simulink model "DroneOptimalPlanning"  (R2020b)
settings: Solver=FixedStepAuto  StartTime=0.0  StopTime=Ttot  RelTol=1e-3
values from neighbouring files (symbols this model uses):
  A = eval(A)    [Pianificazione1.m]
  A_d_fe = Ts*A + eye(size(A,1))    [Pianificazione1.m]
  A_d_zoh = sys_d_zoh.a    [Pianificazione1.m]
  B = eval(B)    [Pianificazione1.m]
  B_d_fe = Ts*B    [Pianificazione1.m]
  B_d_zoh = sys_d_zoh.b    [Pianificazione1.m]
  C = eye(12)    [Pianificazione1.m]
  C_d_fe = C    [Pianificazione1.m]
  C_d_zoh = sys_d_zoh.c    [Pianificazione1.m]
  D = zeros(12,4)    [Pianificazione1.m]
  D_d_fe = D    [Pianificazione1.m]
  D_d_zoh = sys_d_zoh.d    [Pianificazione1.m]
  F_lb = -6/4    (= -1.5)    [Pianificazione1.m]
  F_ub = 2    [Pianificazione1.m]
  Ts = 0.1    [Pianificazione1.m]
  x_0 = [0;0;0;0;0;0;0;0;0;0;0;0]    [Pianificazione1.m]
settings Model: Creator=Tommaso  LastModifiedBy=Tommaso
settings OptimizationCC: DefaultParameterBehavior=Inlined  UseDivisionForNetSlopeComputation=on  GainParamInheritBuiltInType=on  UseFloatMulNetSlope=on  InlineInvariantSignals=on  PassReuseOutputArgsAs=Individual arguments  ZeroExternalMemoryAtStartup=off  ZeroInternalMemoryAtStartup=off  NoFixptDivByZeroProtection=on  EfficientFloat2IntCast=on  LifeSpan=1  OptimizeBlockOrder=speed  DifferentSizesBufferReuse=on  EfficientTunableParamExpr=on
settings DebuggingCC: ParameterTunabilityLossMsg=error
settings HardwareCC: ProdBitPerPointer=32  ProdBitPerSizeT=32  ProdBitPerPtrDiffT=32  ProdLargestAtomicInteger=Long  ProdLargestAtomicFloat=Double  ProdWordSize=32  ProdLongLongMode=on  ProdHWDeviceType=ARM Compatible->ARM Cortex-M
settings SFSimCC: MATLABDynamicMemAlloc=off
settings RTWCC: Description=Embedded Coder  SystemTargetFile=ert.tlc  TemplateMakefile=ert_default_tmf  TargetLang=C++
settings CodeAppCC: ForceParamTrailComments=on  IgnoreCustomStorageClasses=off  OperatorAnnotations=on  SimulinkDataObjDesc=on  SFDataObjDesc=on  CustomSymbolStrGlobalVar=rt$N$M  CustomSymbolStrType=$N$M  CustomSymbolStrFcn=$N$M$F  CustomSymbolStrMacro=$N$M  InsertBlockDesc=on
settings ERTTargetCC: TargetLangStandard=C++03 (ISO)  GenerateSampleERTMain=on  IncludeMdlTerminateFcn=off  CombineSignalStateStructs=on  CodeInterfacePackaging=C++ class  SupportComplex=off  SupportContinuousTime=on  InlinedParameterPlacement=NonHierarchical  RootIOFormat=Structure reference  ERTCustomFileTemplate=example_file_process.tlc  ERTFilePackagingFormat=CompactWithDataFile

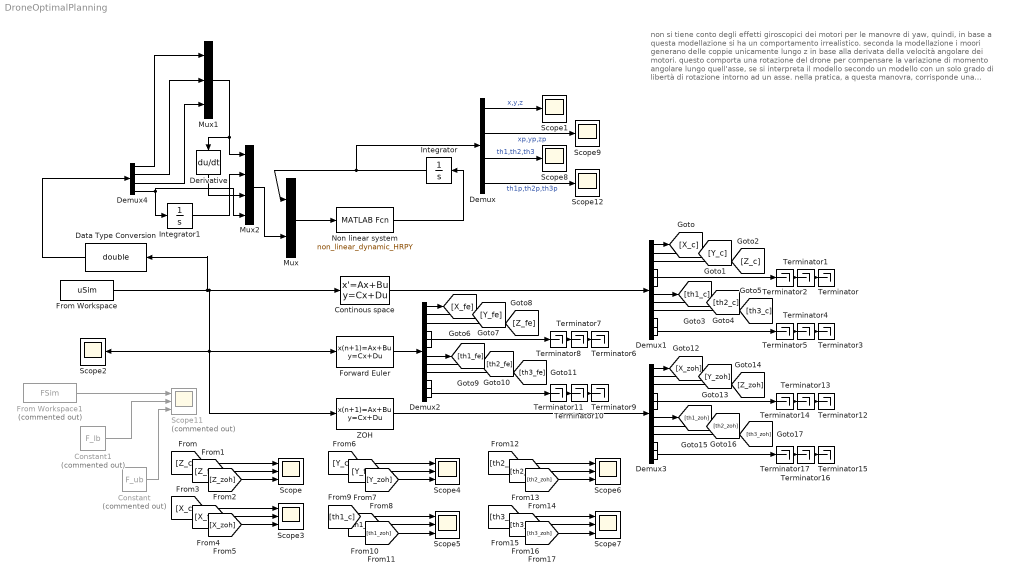
== system DroneOptimalPlanning ==
  note: non si tiene conto degli effetti giroscopici dei motori per le manovre
      | di yaw, quindi, in base a questa modellazione si ha un comportamento irrealistico.
      | seconda la modellazione i moori generano delle coppie unicamente lungo z in base
      | alla derivata della velocità angolare dei motori. questo comporta una rotazione del drone
      | per compensare la variazione di momento angolare lungo quell'asse, se si interpreta il modello secondo un modello con un solo grado di libertà di rotazione intorno ad un asse.
      | nella pratica, a questa manovra, corrisponde una variazione del momento angolare dei motori a cui si accompagna un effetto giroscopico. questi aspetti non sono stati
      | approfonditi. Per incldere quesi aspetti nella modellazione sarebbe necessario modellare
      | la dinamica dei motori e considerare che questi siano montati sul riferimento body
      | a quel punto subentrebbero nelle equazioni degli accoppiamenti tra omegab_x
      | e omegam_z
      | Ho modellato solo l'effetto giroscopico del drone come oggetto nello spazio
      | ho trascurato l'effetto giroscopico dei motori, che è nullo per tutte le manovre
      | ma non per l'imbardata
  Constant : Constant  Commented=on  Value=F_ub
  Constant1 : Constant  Commented=on  Value=F_lb
  Continous space : StateSpace  A=A  B=B  C=C  D=D  InitialCondition=x_0
  Data Type Conversion : DataTypeConversion  OutDataTypeStr=double
  Demux : Demux
  Demux1 : Demux  Outputs=12
  Demux2 : Demux  Outputs=12
  Demux3 : Demux  Outputs=12
  Demux4 : Demux
  Derivative : Derivative
  Forward Euler : DiscreteStateSpace  A=A_d_fe  B=B_d_fe  C=C_d_fe  D=D_d_fe  InitialCondition=x_0  SampleTime=Ts
  From Workspace : FromWorkspace  VariableName=uSim  SampleTime=Ts  OutputAfterFinalValue=Holding final value
  From Workspace1 : FromWorkspace  Commented=on  VariableName=FSim  SampleTime=Ts  OutputAfterFinalValue=Holding final value
  Integrator : Integrator  InitialCondition=x_0  LimitOutput=on  UpperSaturationLimit=10^6  LowerSaturationLimit=-10^6
  Integrator1 : Integrator
  Mux : Mux  Inputs=2
  Mux1 : Mux  Inputs=3
  Mux2 : Mux
  Non linear system : MATLABFcn  MATLABFcn=non_linear_dynamic_HRPY
  Scope{,3..7} (6 alike) : Scope  NumInputPorts=3
  Scope{1..2,8..9,12} (5 alike) : Scope
  Scope11 : Scope  Commented=on  NumInputPorts=3
  Terminator{,1..17} (18 alike) : Terminator
  ZOH : DiscreteStateSpace  A=A_d_zoh  B=B_d_zoh  C=C_d_zoh  D=D_d_zoh  InitialCondition=x_0  SampleTime=Ts
  wires:
  From Workspace/1 -> Data Type Conversion/1, Continous space/1, Scope2/1, ZOH/1, Forward Euler/1
  Mux/1 -> Non linear system/1
  Integrator/1 -> Demux/1, Mux/1
  Non linear system/1 -> Integrator/1
  Continous space/1 -> Demux1/1
  Forward Euler/1 -> Demux2/1
  Demux/1 -> Scope1/1  "x,y,z"
  Demux/3 -> Scope8/1  "th1,th2,th3"
  Demux4/1 -> Mux1/1
  Demux4/2 -> Mux1/2
  Demux4/3 -> Mux1/3
  Demux4/4 -> Mux2/4, Integrator1/1
  Integrator1/1 -> Mux2/2
  Mux1/1 -> Derivative/1, Mux2/1
  Derivative/1 -> Mux2/3
  Mux2/1 -> Mux/2
  Demux/2 -> Scope9/1  "xp,yp,zp"
  From Workspace1/1 -> Scope11/1
  Constant1/1 -> Scope11/2
  Constant/1 -> Scope11/3
  Data Type Conversion/1 -> Demux4/1
  Demux/4 -> Scope12/1  "th1p,th2p,th3p"
  Demux1/1 -> [X_c]
  Demux1/2 -> [Y_c]
  Demux1/3 -> [Z_c]
  Demux1/7 -> [th1_c]
  Demux1/8 -> [th2_c]
  Demux1/9 -> [th3_c]
  Demux1/5 -> Terminator1/1
  Demux1/6 -> Terminator/1
  Demux1/4 -> Terminator2/1
  [Z_c] -> Scope/1
  [Z_fe] -> Scope/2
  [Z_zoh] -> Scope/3
  [X_c] -> Scope3/1
  [X_zoh] -> Scope3/3
  [X_fe] -> Scope3/2
  [Y_c] -> Scope4/1
  [Y_zoh] -> Scope4/3
  [Y_fe] -> Scope4/2
  [th1_c] -> Scope5/1
  [th1_zoh] -> Scope5/3
  [th1_fe] -> Scope5/2
  [th2_c] -> Scope6/1
  [th2_zoh] -> Scope6/3
  [th2_fe] -> Scope6/2
  [th3_c] -> Scope7/1
  [th3_zoh] -> Scope7/3
  [th3_fe] -> Scope7/2
  Demux1/10 -> Terminator5/1
  Demux1/11 -> Terminator4/1
  Demux1/12 -> Terminator3/1
  Demux2/5 -> Terminator7/1
  Demux2/4 -> Terminator8/1
  Demux2/11 -> Terminator10/1
  Demux2/10 -> Terminator11/1
  Demux2/9 -> [th3_fe]
  Demux2/8 -> [th2_fe]
  Demux2/7 -> [th1_fe]
  Demux2/2 -> [Y_fe]
  Demux2/1 -> [X_fe]
  Demux2/3 -> [Z_fe]
  Demux2/6 -> Terminator6/1
  Demux2/12 -> Terminator9/1
  Demux3/5 -> Terminator13/1
  Demux3/4 -> Terminator14/1
  Demux3/11 -> Terminator16/1
  Demux3/10 -> Terminator17/1
  Demux3/9 -> [th3_zoh]
  Demux3/8 -> [th2_zoh]
  Demux3/7 -> [th1_zoh]
  Demux3/2 -> [Y_zoh]
  Demux3/1 -> [X_zoh]
  Demux3/3 -> [Z_zoh]
  Demux3/6 -> Terminator12/1
  Demux3/12 -> Terminator15/1
  ZOH/1 -> Demux3/1
